simulink library "Isolated_Cover"  (R2018b)
settings: Solver=ode45  StartTime=0.0  StopTime=10.0  RelTol=1e-3  EnableMultiTasking=on
settings Model: Creator=lena.frank  LastModifiedBy=P41573
settings DataIOCC: LimitDataPoints=on  SaveFormat=Array  SignalLoggingSaveFormat=ModelDataLogs
settings OptimizationCC: ExpressionDepthLimit=2147483647  LifeSpan=inf
settings DebuggingCC: UnderspecifiedInitializationDetection=Classic  MergeDetectMultiDrivingBlocksExec=none  SolverPrmCheckMsg=warning  FcnCallInpInsideContextMsg=warning  StateNameClashWarn=warning  SFUnexpectedBacktrackingDiag=warning  SFNoUnconditionalDefaultTransitionDiag=warning  SFExecutionAtInitializationDiag=none
settings HardwareCC: ProdBitPerPointer=32  ProdBitPerSizeT=32  ProdBitPerPtrDiffT=32  ProdLargestAtomicFloat=None  ProdIntDivRoundTo=Undefined  ProdEndianess=Unspecified  ProdWordSize=32  ProdHWDeviceType=32-bit Generic
settings ModelReferenceCC: PropagateSignalLabelsOutOfModel=off
settings SFSimCC: SimUseLocalCustomCode=off
settings RTWCC: RTWUseLocalCustomCode=off
settings CodeAppCC: StateflowObjectComments=on
settings GRTTargetCC: TargetLangStandard=C89/C90 (ANSI)  GeneratePreprocessorConditionals=Disable all  CombineOutputUpdateFcns=off  GRTInterface=on
settings ConfigComp: CovMetricSettings=dw  CovHtmlReporting=on  CovSaveCumulativeToWorkspaceVar=on  CovSaveSingleToWorkspaceVar=on  CovExternalEMLEnable=off

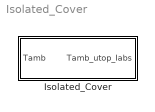
== system Isolated_Cover ==
  Isolated_Cover : Subsystem  mask(isolated cover){u=0.6}
      mask prompts: u "loss coefficient of isolation [W/(m²*K)]"
      mask help: This is a surface-model for ground storages. It describes the absorption of solar radiation and the heat losses by wind.
      mask Help: web(fullfile(path_carnot('help'),'Isolated_Cover.html'),'-helpbrowser')

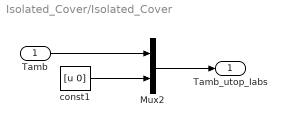
== system Isolated_Cover/Isolated_Cover ==
  Tamb : Inport
  Mux2 : Mux  Inputs=2
  const1 : Constant  Value=[u 0]
  Tamb_utop_Iabs : Outport
  wires:
  Tamb/1 -> Mux2/1
  const1/1 -> Mux2/2
  Mux2/1 -> Tamb_utop_Iabs/1
